simulink model "adaptive_force_control_0111_backup"  (R2022b)
settings: Solver=daessc  StartTime=0.0  StopTime=5  FixedStep=0.0005  MaxStep=0.0025  RelTol=2e-2  AbsTol=2e-2  EnableMultiTasking=on
StopFcn:
  | Initialize = 0;
model workspace (MAT data in the model file):
  Initialize : Simulink.Signal (value not decoded)
  Var = [0; 0; 0]
values from neighbouring files (symbols this model uses):
  joint_kd = 1.75    [simulink_param.m]
  joint_ki = 0.8    [simulink_param.m]
  joint_kp = 60    [simulink_param.m]
undefined symbols (not defined in the file or in its folder): X, Y, Z
libraries: sm_lib x86, nesl_utility x22, simulink x8, fl_lib x8, slpidlib x4, eeGeneralControl x3, Contact_Forces_Lib x1
(part 4 of 4)

== system adaptive_force_control_0111_backup/Subsystem2/joint_G ==
  jointG : sm_lib/Joints/Bearing Joint  JointMode=Normal  SenseConstraintForce=off  SenseConstraintForceX=off  SenseConstraintForceY=off  SenseConstraintForceZ=off  SenseConstraintTorque=off  SenseConstraintTorqueX=off  SenseConstraintTorqueY=off  SenseConstraintTorqueZ=off  SenseTotalForce=off  SenseTotalForceX=off  SenseTotalForceY=off  SenseTotalForceZ=off  SenseTotalTorque=off  SenseTotalTorqueX=off  SenseTotalTorqueY=off  SenseTotalTorqueZ=off  CompositeWrenchDir=FollowerOnBase  CompositeWrenchFrame=BaseFrame  PzEquilibriumPosition=0  PzEquilibriumPositionUnits=m  PzSpringStiffness=0  PzSpringStiffnessUnits=N/m  PzDampingCoefficient=0  PzDampingCoefficientUnits=N/(m/s)  PzTorqueActuationMode=NoTorque  PzMotionActuationMode=ComputedMotion  PzSensePosition=off  PzSenseVelocity=off  PzSenseAcceleration=off  PzSenseTorqueForce=off  PzSenseLowerLimitTorqueForce=off  PzSenseUpperLimitTorqueForce=off  PzLowerLimitSpecify=off  PzLowerLimitBound=-1  PzLowerLimitBoundUnits=m  PzLowerLimitStiffness=1e6  PzLowerLimitStiffnessUnits=N/m  PzLowerLimitDamping=1e3  PzLowerLimitDampingUnits=N/(m/s)  PzLowerLimitTransitionRegionWidth=1e-4  PzLowerLimitTransitionRegionWidthUnits=m  PzUpperLimitSpecify=off  PzUpperLimitBound=1  PzUpperLimitBoundUnits=m  PzUpperLimitStiffness=1e6  PzUpperLimitStiffnessUnits=N/m  PzUpperLimitDamping=1e3  PzUpperLimitDampingUnits=N/(m/s)  PzUpperLimitTransitionRegionWidth=1e-4  PzUpperLimitTransitionRegionWidthUnits=m  PzPositionTargetSpecify=off  PzPositionTargetPriority=High  PzPositionTargetValue=0  PzPositionTargetValueUnits=m  PzVelocityTargetSpecify=off  PzVelocityTargetPriority=High  PzVelocityTargetValue=0  PzVelocityTargetValueUnits=m/s  RxEquilibriumPosition=0  RxEquilibriumPositionUnits=deg  RxSpringStiffness=0  RxSpringStiffnessUnits=N*m/deg  RxDampingCoefficient=0  RxDampingCoefficientUnits=N*m/(deg/s)  RxTorqueActuationMode=NoTorque  RxMotionActuationMode=ComputedMotion  RxSensePosition=off  RxSenseVelocity=off  RxSenseAcceleration=off  RxSenseTorqueForce=off  RxSenseLowerLimitTorqueForce=off  RxSenseUpperLimitTorqueForce=off  RxLowerLimitSpecify=off  RxLowerLimitBound=-90  RxLowerLimitBoundUnits=deg  RxLowerLimitStiffness=1e4  RxLowerLimitStiffnessUnits=N*m/deg  RxLowerLimitDamping=10  RxLowerLimitDampingUnits=N*m/(deg/s)  RxLowerLimitTransitionRegionWidth=0.1  RxLowerLimitTransitionRegionWidthUnits=deg  RxUpperLimitSpecify=off  RxUpperLimitBound=90  RxUpperLimitBoundUnits=deg  RxUpperLimitStiffness=1e4  RxUpperLimitStiffnessUnits=N*m/deg  RxUpperLimitDamping=10  RxUpperLimitDampingUnits=N*m/(deg/s)  RxUpperLimitTransitionRegionWidth=0.1  RxUpperLimitTransitionRegionWidthUnits=deg  RxPositionTargetSpecify=off  RxPositionTargetPriority=High  RxPositionTargetValue=0  RxPositionTargetValueUnits=deg  RxVelocityTargetSpecify=off  RxVelocityTargetPriority=High  RxVelocityTargetValue=0  RxVelocityTargetValueUnits=deg/s  RyEquilibriumPosition=0  RyEquilibriumPositionUnits=deg  RySpringStiffness=0  RySpringStiffnessUnits=N*m/deg  RyDampingCoefficient=0  RyDampingCoefficientUnits=N*m/(deg/s)  RyTorqueActuationMode=NoTorque  RyMotionActuationMode=ComputedMotion  RySensePosition=off  RySenseVelocity=off  RySenseAcceleration=off  RySenseTorqueForce=off  RySenseLowerLimitTorqueForce=off  RySenseUpperLimitTorqueForce=off  RyLowerLimitSpecify=off  RyLowerLimitBound=-90  RyLowerLimitBoundUnits=deg  RyLowerLimitStiffness=1e4  RyLowerLimitStiffnessUnits=N*m/deg  RyLowerLimitDamping=10  RyLowerLimitDampingUnits=N*m/(deg/s)  RyLowerLimitTransitionRegionWidth=0.1  RyLowerLimitTransitionRegionWidthUnits=deg  RyUpperLimitSpecify=off  RyUpperLimitBound=90  RyUpperLimitBoundUnits=deg  RyUpperLimitStiffness=1e4  RyUpperLimitStiffnessUnits=N*m/deg  RyUpperLimitDamping=10  RyUpperLimitDampingUnits=N*m/(deg/s)  RyUpperLimitTransitionRegionWidth=0.1  RyUpperLimitTransitionRegionWidthUnits=deg  RyPositionTargetSpecify=off  RyPositionTargetPriority=High  RyPositionTargetValue=0  RyPositionTargetValueUnits=deg  RyVelocityTargetSpecify=off  RyVelocityTargetPriority=High  RyVelocityTargetValue=0  RyVelocityTargetValueUnits=deg/s  RzEquilibriumPosition=0  RzEquilibriumPositionUnits=deg  RzSpringStiffness=0  RzSpringStiffnessUnits=N*m/deg  RzDampingCoefficient=0  RzDampingCoefficientUnits=N*m/(deg/s)  RzTorqueActuationMode=NoTorque  RzMotionActuationMode=ComputedMotion  RzSensePosition=off  RzSenseVelocity=off  RzSenseAcceleration=off  RzSenseTorqueForce=off  RzSenseLowerLimitTorqueForce=off  RzSenseUpperLimitTorqueForce=off  RzLowerLimitSpecify=off  RzLowerLimitBound=-90  RzLowerLimitBoundUnits=deg  RzLowerLimitStiffness=1e4  RzLowerLimitStiffnessUnits=N*m/deg  RzLowerLimitDamping=10  RzLowerLimitDampingUnits=N*m/(deg/s)  RzLowerLimitTransitionRegionWidth=0.1  RzLowerLimitTransitionRegionWidthUnits=deg  RzUpperLimitSpecify=off  RzUpperLimitBound=90  RzUpperLimitBoundUnits=deg  RzUpperLimitStiffness=1e4  RzUpperLimitStiffnessUnits=N*m/deg  RzUpperLimitDamping=10  RzUpperLimitDampingUnits=N*m/(deg/s)  RzUpperLimitTransitionRegionWidth=0.1  RzUpperLimitTransitionRegionWidthUnits=deg  RzPositionTargetSpecify=off  RzPositionTargetPriority=High  RzPositionTargetValue=0  RzPositionTargetValueUnits=deg  RzVelocityTargetSpecify=off  RzVelocityTargetPriority=High  RzVelocityTargetValue=0  RzVelocityTargetValueUnits=deg/s
  long_pin : sm_lib/Body Elements/File Solid  ExtGeomFileName=./CAD/MBD_long_pin.stl  UnitType=Custom  ExtGeomFileUnits=mm  StepReaderType=HEX  ExportConvexHullGeometry=off  InertiaType=CalculateFromGeometry  Mass=11  MassUnits=g  CenterOfMass=[0 0 0]  CenterOfMassUnits=m  MomentsOfInertia=[1 1 1]  MomentsOfInertiaUnits=kg*m^2  ProductsOfInertia=[0 0 0]  ProductsOfInertiaUnits=kg*m^2  BasedOnType=Mass  Density=1000  DensityUnits=kg/m^3  DoExposeReferenceFrame=on  SerializedFrames=<Frames/>  GraphicType=FromGeometry  MarkerShape=Sphere  MarkerSize=10  GraphicVisPropType=SimpleVisualProperties  GraphicDiffuseColor=[0.5 0.5 0.5]  GraphicSpecularColor=[0.5 0.5 0.5 1.0]  GraphicAmbientColor=[0.15 0.15 0.15 1.0]  GraphicEmissiveColor=[0.0 0.0 0.0 1.0]  GraphicShininess=75  GraphicOpacity=1.0
  Conn1 : PMIOPort  Side=Left
  Conn2 : PMIOPort  Port=2  Side=Left
  connections:
  long_pin/RConn1 -- Conn1/RConn1 -- jointG/RConn1
  jointG/LConn1 -- Conn2/RConn1

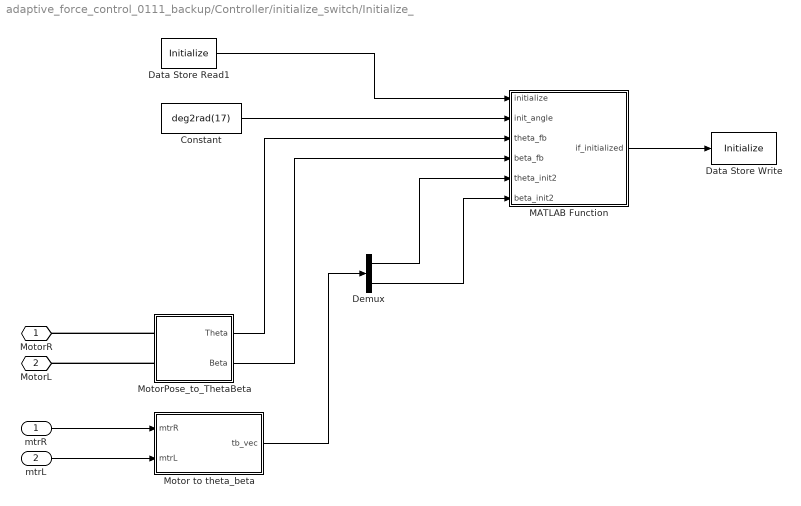
== system adaptive_force_control_0111_backup/Controller/initialize_switch/Initialize_ ==
  mtrR : Inport
  mtrL : Inport  Port=2
  Constant : Constant  Value=deg2rad(17)
  Data Store Read1 : DataStoreRead  DataStoreName=Initialize  IndexOptions=Index vector (dialog)  Indices=1  OutputSizes=1
  Data Store Write : DataStoreWrite  DataStoreName=Initialize  IndexOptions=Index vector (dialog)  Indices=1  OutputSizes=1
  Demux : Demux  Outputs=2
  MATLAB Function : MATLAB Function  TreatAsAtomicUnit=on
  Motor to theta_beta : MATLAB Function  TreatAsAtomicUnit=on
  MotorPose_to_ThetaBeta : Subsystem
  MotorR : PMIOPort  Side=Left
  MotorL : PMIOPort  Port=2  Side=Left
  wires:
  MATLAB Function/1(if_initialized) -> Data Store Write/1
  Data Store Read1/1 -> MATLAB Function/1(initialize)
  MotorPose_to_ThetaBeta/1(Theta) -> MATLAB Function/3(theta_fb)
  Constant/1 -> MATLAB Function/2(init_angle)
  MotorPose_to_ThetaBeta/2(Beta) -> MATLAB Function/4(beta_fb)
  mtrL/1 -> Motor to theta_beta/2(mtrL)
  mtrR/1 -> Motor to theta_beta/1(mtrR)
  Motor to theta_beta/1(tb_vec) -> Demux/1
  Demux/1 -> MATLAB Function/5(theta_init2)
  Demux/2 -> MATLAB Function/6(beta_init2)
  connections:
  MotorPose_to_ThetaBeta/LConn2 -- MotorL/RConn1
  MotorPose_to_ThetaBeta/LConn1 -- MotorR/RConn1

== system adaptive_force_control_0111_backup/Controller/initialize_switch/Initialize_/MotorPose_to_ThetaBeta ==
  Demux : Demux  Outputs=2
  Motor to theta_beta1 : MATLAB Function  TreatAsAtomicUnit=on
  PS-Simulink Converter1 : nesl_utility/PS-Simulink Converter  PhysicalDomain=network_engine_domain  SubClassName=ps_output  LeftPortType=input  RightPortType=output  PseudoPeriodic=off  Frequencies=[]  VectorFormat=inherit  Unit=inherit  AffineConversion=off
  PS-Simulink Converter2 : nesl_utility/PS-Simulink Converter  PhysicalDomain=network_engine_domain  SubClassName=ps_output  LeftPortType=input  RightPortType=output  PseudoPeriodic=off  Frequencies=[]  VectorFormat=inherit  Unit=inherit  AffineConversion=off
  MotorR : PMIOPort  Side=Left
  MotorL : PMIOPort  Port=2  Side=Left
  Theta : Outport
  Beta : Outport  Port=2
  wires:
  Motor to theta_beta1/1(tb_vec) -> Demux/1
  Demux/1 -> Theta/1
  PS-Simulink Converter1/1 -> Motor to theta_beta1/1(mtrR)
  PS-Simulink Converter2/1 -> Motor to theta_beta1/2(mtrL)
  Demux/2 -> Beta/1
  connections:
  MotorR/RConn1 -- PS-Simulink Converter1/LConn1
  MotorL/RConn1 -- PS-Simulink Converter2/LConn1

== matlab function adaptive_force_control_0111_backup/Controller/SimMotorPose_to_ThetaBeta/Motor to theta_beta ==
  data: mtrR input; tb_vec output; mtrL input
function tb_vec = Mtr_to_tb(mtrR, mtrL)
phi_vec = [pi/2 - mtrR; pi/2 - mtrL];

R = pi/2 - mtrR;
L = pi/2 - mtrL;

r = exp(R*i);
l = exp(L*i);
theta = angle(r/l);
if theta < 0
    theta = theta + 2*pi;
end

theta = theta/2;
beta = angle(l) + theta;
tb_vec = [theta; beta];

% tb_vec = 1/2 * [1 -1; 1 1]*phi_vec;

== matlab function adaptive_force_control_0111_backup/Controller/initialize_switch/Initialize_/MATLAB Function ==
  data: initialize input; init_angle input; theta_fb input; if_initialized output; beta_fb input; theta_init2 input; beta_init2 input
function if_initialized = fcn(initialize, init_angle, theta_fb, beta_fb, theta_init2, beta_init2)
% if initialize == 0
%     if abs(theta - init_angle) < 0.01
%         if_initialized = 1;
%     else
%         if_initialized = 0;
%     end
% else
%     if_initialized = 1;
% end

if initialize == 0
    if abs(theta_fb - init_angle) < 0.01
        if_initialized = 1;
    else
        if_initialized = 0;
    end
elseif initialize == 1
    if abs(beta_fb-beta_init2) < 0.03 && abs(theta_fb-theta_init2) < 0.03
        if_initialized = 2;    
    else
        if_initialized = 1;
    end
elseif initialize == 2
    if_initialized = 2;
else
    if_initialized = 0;
end

% if initialize == 1
%     if abs(beta) < 0.01
%         if_initialized =2 ;
%     else
%         if_initialized=1;
%     end
% else
%     if_initialized=1;
% end
% disp(beta)
% disp(if_initialized)

end

== matlab function adaptive_force_control_0111_backup/Controller/IK1 ==
  data: xy input; tb output
function tb = inverse_kinematics(xy)
x = xy(1);
y = xy(2);
ik_pc_ = [4.10837754e+05, -6.25071622e+05, 4.02616603e+05, -1.41754291e+05, 2.93469460e+04, -3.56228405e+03, 2.44240485e+02, -7.12383946e+00];
L = sqrt(x^2 + y^2);
theta = polyval(ik_pc_, L);
u_xy = [x, y]/L;
beta = acos(-u_xy*[0;1]);
beta = abs(beta) * sign(x)*(-1);
tb = [theta, beta];

== matlab function adaptive_force_control_0111_backup/R_joint/MATLAB Function ==
  data: w input; T_friction output; t input
function T_friction = fcn(w, t)
% Friction model by Y.C. exp.
% input: angular velocity and actuation torque of motor
% Coeff.
p00 = -0.3321;
p10 = 0.02744;
p01 = -0.02039;
p20 = -0.00691;
p11 = -0.01989;
p02 = -0.001946;
p30 = 0.0006073;
p21 = 0.003026;
p12 = 0.0006086;
p40 = -1.75e-05;
p31 = -9.304e-05;
p22 = -5.24e-05;

X = w;
Y = t;
Z = p00 + p10.*X + p01.*Y + p20.*(X.^2) + p11.*X.*Y + p02.*(Y.^2) + p30.*(X.^3) + p21.*(X.^2).*Y + p12.*X.*(Y.^2) + p40.*(X.^4) + p31.*(X.^3).*Y + p22.*(X.^2).*(Y.^2);

T_friction = Z;

== matlab function adaptive_force_control_0111_backup/Controller/MATLAB Function2 ==
  data: ThetaBeta input; SimPhiRL output
function SimPhiRL = getSimPhiRL(ThetaBeta)
tb = reshape(ThetaBeta, [2,1]);
PhiRL = [1 1; -1 1]* tb - [1; -1]*deg2rad(17);
SimPhiRL = [deg2rad(90-17) - PhiRL(1), deg2rad(90+17) - PhiRL(2)];
end

== matlab function adaptive_force_control_0111_backup/Controller/IK ==
  data: xy input; tb output
function tb = inverse_kinematics(xy)
x = xy(1);
y = xy(2);
ik_pc_ = [4.10837754e+05, -6.25071622e+05, 4.02616603e+05, -1.41754291e+05, 2.93469460e+04, -3.56228405e+03, 2.44240485e+02, -7.12383946e+00];
L = sqrt(x^2 + y^2);
theta = polyval(ik_pc_, L);
u_xy = [x, y]/L;
beta = acos(-u_xy*[0;1]);

tb = [theta, beta];

== matlab function adaptive_force_control_0111_backup/Controller/MATLAB Function ==
  data: ThetaBeta input; SimPhiRL output
function SimPhiRL = getSimPhiRL(ThetaBeta)
tb = reshape(ThetaBeta, [2,1]);
PhiRL = [1 1; -1 1]* tb - [1; -1]*deg2rad(17);
SimPhiRL = [deg2rad(90-17) - PhiRL(1), deg2rad(90+17) - PhiRL(2)];
end

== matlab function adaptive_force_control_0111_backup/Controller/initialize_switch/Initialize_/Motor to theta_beta ==
  data: mtrR input; tb_vec output; mtrL input
function tb_vec = Mtr_to_tb(mtrR, mtrL)
phi_vec = [pi/2 - mtrR; pi/2 - mtrL];
tb_vec = 1/2 * [1 -1; 1 1]*phi_vec;

== matlab function adaptive_force_control_0111_backup/Controller/initialize_switch/Initialize_/MotorPose_to_ThetaBeta/Motor to theta_beta1 ==
  data: mtrR input; tb_vec output; mtrL input
function tb_vec = Mtr_to_tb(mtrR, mtrL)
phi_vec = [pi/2 - mtrR; pi/2 - mtrL];
tb_vec = 1/2 * [1 -1; 1 1]*phi_vec;
